simulink model "vehicles"  (Simulink 6.5)
settings: Solver=ode45  StartTime=0.0  StopTime=50  FixedStep=.1  RelTol=1e-3
PreLoadFcn:
  | vehicledata; % load in workspace variables
  | h=frontend; % bring up GUI
  | movegui(h,'northwest') % move gui to top right
PostLoadFcn:
  | rt=sfroot; chart=rt.find('-isa', 'Stateflow.Chart', '-and', 'Name','uav_modes'); chart.view;
undefined symbols (not defined in the file or in its folder): Cd0, Clmax, Clmin, g, initthis, k, magnitude, mat2cell, num_ac, num_instincts, obstacles, omega_chi, omega_gamma, omega_v, rho, S, sigma_a, sigma_o, sigma_t1, sigma_t2, targets, Tmax, W
libraries: dspmtrx3 x38, dspindex x5, dspstat3 x4, vrlib x2
(part 1 of 2)
settings Model: Creator=dlluch  LastModifiedBy=dlluch  BufferReuse=off
settings DataIOCC: LimitDataPoints=off  SaveOutput=off  SaveState=on  SignalLoggingName=sigsOut
settings OptimizationCC: BooleanDataType=off  InlineInvariantSignals=on  OptimizeBlockIOStorage=off  BufferReuse=off  ExpressionFolding=off  LocalBlockOutputs=off
settings DebuggingCC: SolverPrmCheckMsg=none  MultiTaskDSMMsg=warning  MultiTaskCondExecSysMsg=none  UnconnectedInputMsg=none  UnconnectedOutputMsg=none  UnconnectedLineMsg=none  StrictBusMsg=None
settings HardwareCC: TargetUnknown=on
settings RTWCC: IncludeERTFirstTime=on

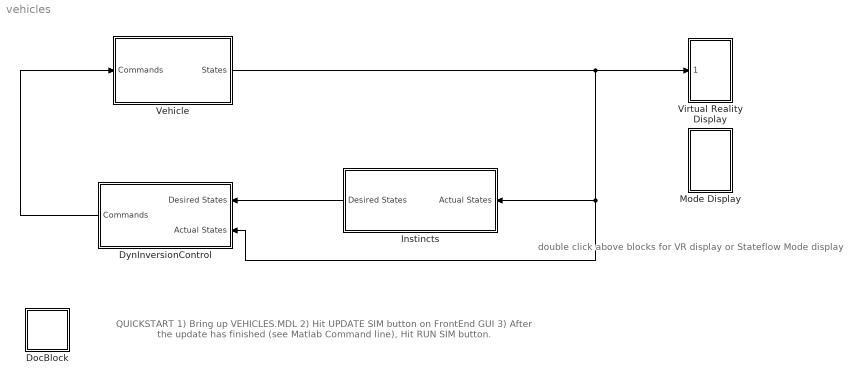
== system vehicles ==
  note: QUICKSTART
      | 1) Bring up VEHICLES.MDL
      | 2) Hit UPDATE SIM button on FrontEnd GUI
      | 3) After the update has finished (see Matlab Command line), Hit RUN SIM button.
  note: double click above
      | blocks for VR display
      | or Stateflow Mode
      | display
  DocBlock : Subsystem  mask(DocBlock){ECoderFlag=, DocumentType=Text}
      mask prompts: ECoderFlag "E Coder Flag"; DocumentType "Document Type"
      mask help: Use this block to save long descriptive text with the model. Double-clicking the block will open an editor.
      settings: CopyFcn=docblock('breaklink',gcb);  DeleteFcn=docblock('close_document',gcb);  PreSaveFcn=docblock('save_document',gcb);  OpenFcn=docblock('edit_document',gcb);
      mask StyleString: edit,popup(Text|RTF|HTML)
      mask Display:
      | plot([.8 0 0 1 1 .8 .8 1],[1 1 0 0 .8 1 .8 .8]);
      | text(.5,.5,'DOC','horizontalalignment','center');
  DynInversionControl : Subsystem  Orientation=left
  Instincts : Subsystem  Orientation=left
  Mode Display : Subsystem
      settings: OpenFcn=rt=sfroot; chart=rt.find('-isa', 'Stateflow.Chart', '-and', '-regexp', 'Name','uav_modes'); chart.view;
  Vehicle : Subsystem
  Virtual Reality Display : Subsystem
      settings: OpenFcn=|
      | h_vrsink=find_system(gcbh,'referenceblock','vrlib/VR Sink')
      | vrmfunc('FnOpen', h_vrsink);
  wires:
  Vehicle/1(States) -> Instincts/1(Actual States), DynInversionControl/2(Actual States), Virtual Reality Display/1(States)
  Instincts/1(Desired States) -> DynInversionControl/1(Desired States)
  DynInversionControl/1(Commands) -> Vehicle/1(Commands)

== system vehicles/DocBlock ==
  EmptySubsystem : Subsystem

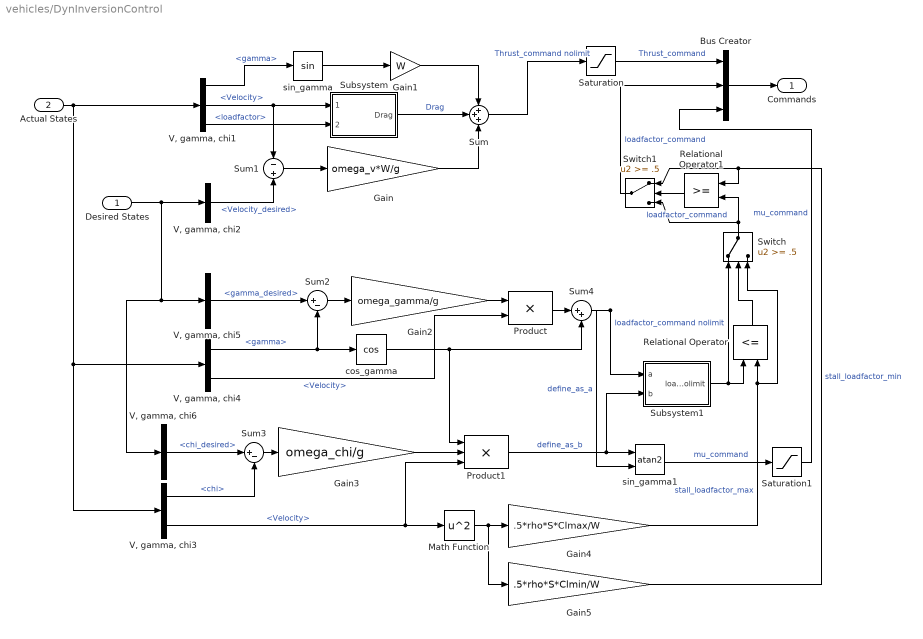
== system vehicles/DynInversionControl ==
  Desired States : Inport
  Actual States : Inport  Port=2
  Bus Creator : BusCreator  Inputs=3
  Gain : Gain  Gain=omega_v*W/g  SaturateOnIntegerOverflow=on
  Gain1 : Gain  Gain=W  SaturateOnIntegerOverflow=on
  Gain2 : Gain  Gain=omega_gamma/g  SaturateOnIntegerOverflow=on
  Gain3 : Gain  Gain=omega_chi/g  SaturateOnIntegerOverflow=on
  Gain4 : Gain  Gain=.5*rho*S*Clmax/W  SaturateOnIntegerOverflow=on
  Gain5 : Gain  Gain=.5*rho*S*Clmin/W  SaturateOnIntegerOverflow=on
  Math Function : Math  Operator=square  SaturateOnIntegerOverflow=on
  Product : Product  SaturateOnIntegerOverflow=on  InputSameDT=on
  Product1 : Product  Inputs=3  SaturateOnIntegerOverflow=on  InputSameDT=on
  Relational Operator : RelationalOperator  Orientation=up  Operator=<=  InputSameDT=on
  Relational Operator1 : RelationalOperator  Orientation=left  InputSameDT=on
  Saturation : Saturate  UpperLimit=Tmax  LowerLimit=0
  Saturation1 : Saturate  UpperLimit=pi/2  LowerLimit=-pi/2
  Subsystem : Subsystem
  Subsystem1 : Subsystem
  Sum : Sum  Inputs=+++  SaturateOnIntegerOverflow=on  InputSameDT=on
  Sum1 : Sum  Inputs=-|+  SaturateOnIntegerOverflow=on  InputSameDT=on
  Sum2 : Sum  Inputs=|+-  SaturateOnIntegerOverflow=on  InputSameDT=on
  Sum3 : Sum  Inputs=|+-  SaturateOnIntegerOverflow=on  InputSameDT=on
  Sum4 : Sum  Inputs=|++  SaturateOnIntegerOverflow=on  InputSameDT=on
  Switch : Switch  Orientation=up  Threshold=.5  SaturateOnIntegerOverflow=on  InputSameDT=on
  Switch1 : Switch  Orientation=left  Threshold=.5  SaturateOnIntegerOverflow=on  InputSameDT=on
  "V, gamma, chi1" : BusSelector  OutputSignals=gamma,Velocity,loadfactor
  "V, gamma, chi2" : BusSelector  OutputSignals=Velocity_desired
  "V, gamma, chi3" : BusSelector  OutputSignals=chi,Velocity
  "V, gamma, chi4" : BusSelector  OutputSignals=gamma,Velocity
  "V, gamma, chi5" : BusSelector  OutputSignals=gamma_desired
  "V, gamma, chi6" : BusSelector  OutputSignals=chi_desired
  cos_gamma : Trigonometry  Operator=cos
  sin_gamma : Trigonometry
  sin_gamma1 : Trigonometry  Operator=atan2
  Commands : Outport
  wires:
  Actual States/1 -> "V, gamma, chi1"/1, "V, gamma, chi3"/1, "V, gamma, chi4"/1
  "V, gamma, chi1"/3 -> Subsystem/2(loadfactor)  "<loadfactor>"
  "V, gamma, chi1"/2 -> Sum1/1, Subsystem/1(Velocity)  "<Velocity>"
  Desired States/1 -> "V, gamma, chi2"/1, "V, gamma, chi5"/1, "V, gamma, chi6"/1
  "V, gamma, chi2"/1 -> Sum1/2  "<Velocity_desired>"
  Sum1/1 -> Gain/1
  Subsystem/1(Drag) -> Sum/2  "Drag"
  Gain/1 -> Sum/3
  "V, gamma, chi1"/1 -> sin_gamma/1  "<gamma>"
  sin_gamma/1 -> Gain1/1
  Gain1/1 -> Sum/1
  Sum/1 -> Saturation/1  "Thrust_command nolimit"
  "V, gamma, chi5"/1 -> Sum2/1  "<gamma_desired>"
  "V, gamma, chi4"/1 -> Sum2/2, cos_gamma/1  "<gamma>"
  "V, gamma, chi6"/1 -> Sum3/1  "<chi_desired>"
  "V, gamma, chi3"/1 -> Sum3/2  "<chi>"
  Sum2/1 -> Gain2/1
  Gain2/1 -> Product/1
  "V, gamma, chi4"/2 -> Product/2  "<Velocity>"
  Product/1 -> Sum4/1
  cos_gamma/1 -> Sum4/2, Product1/1
  Sum4/1 -> sin_gamma1/2, Subsystem1/1(a)  "define_as_a"
  Sum3/1 -> Gain3/1
  Product1/1 -> sin_gamma1/1, Subsystem1/2(b)  "define_as_b"
  sin_gamma1/1 -> Saturation1/1  "mu_command"
  Subsystem1/1(loadfactor_nolimit) -> Switch/1, Relational Operator/1  "loadfactor_command nolimit"
  Bus Creator/1 -> Commands/1
  Saturation/1 -> Bus Creator/1  "Thrust_command"
  "V, gamma, chi3"/2 -> Product1/3, Math Function/1  "<Velocity>"
  Gain3/1 -> Product1/2
  Gain4/1 -> Switch/3, Relational Operator/2  "stall_loadfactor_max"
  Relational Operator/1 -> Switch/2
  Math Function/1 -> Gain4/1, Gain5/1
  Saturation1/1 -> Bus Creator/3  "mu_command"
  Gain5/1 -> Switch1/1, Relational Operator1/1  "stall_loadfactor_min"
  Switch/1 -> Switch1/3, Relational Operator1/2  "loadfactor_command"
  Relational Operator1/1 -> Switch1/2
  Switch1/1 -> Bus Creator/2  "loadfactor_command"

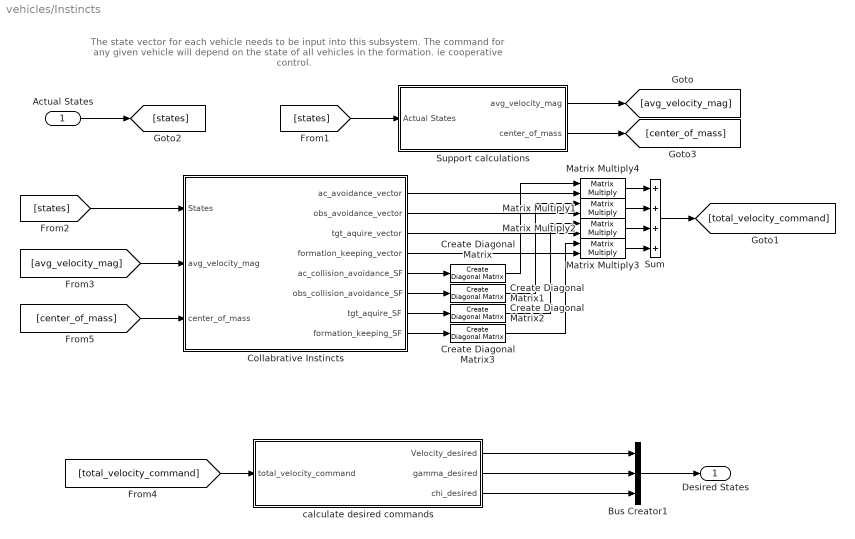
== system vehicles/Instincts ==
  note: The state vector for each vehicle needs to be input into this subsystem.  The command
      | for any given vehicle will depend on the state of all vehicles in the formation.  ie cooperative control.
  Actual States : Inport
  Bus Creator1 : BusCreator  Inputs=3
  Collabrative Instincts : Subsystem
  Create Diagonal Matrix{,1..3} (4 alike) : dspmtrx3/Create Diagonal Matrix
  Matrix Multiply{1..4} (4 alike) : Product  Multiplication=Matrix(*)
  Sum : Sum  Inputs=++++  SaturateOnIntegerOverflow=on  InputSameDT=on
  Support calculations : Subsystem
  calculate desired commands : Subsystem
  Desired States : Outport
  wires:
  Actual States/1 -> [states]
  Support calculations/1(avg_velocity_mag) -> [avg_velocity_mag]
  [states] -> Support calculations/1(Actual States)
  [states] -> Collabrative Instincts/1(States)
  [avg_velocity_mag] -> Collabrative Instincts/2(avg_velocity_mag)
  Support calculations/2(center_of_mass) -> [center_of_mass]
  [center_of_mass] -> Collabrative Instincts/3(center_of_mass)
  Collabrative Instincts/1(ac_avoidance_vector) -> Matrix Multiply4/2
  Collabrative Instincts/2(obs_avoidance_vector) -> Matrix Multiply1/2
  Collabrative Instincts/3(tgt_aquire_vector) -> Matrix Multiply2/2
  Collabrative Instincts/4(formation_keeping_vector) -> Matrix Multiply3/2
  Create Diagonal Matrix/1 -> Matrix Multiply4/1
  Create Diagonal Matrix1/1 -> Matrix Multiply1/1
  Create Diagonal Matrix2/1 -> Matrix Multiply2/1
  Collabrative Instincts/5(ac_collision_avoidance_SF) -> Create Diagonal Matrix/1
  Collabrative Instincts/6(obs_collision_avoidance_SF) -> Create Diagonal Matrix1/1
  Collabrative Instincts/7(tgt_aquire_SF) -> Create Diagonal Matrix2/1
  Collabrative Instincts/8(formation_keeping_SF) -> Create Diagonal Matrix3/1
  Matrix Multiply4/1 -> Sum/1
  Matrix Multiply1/1 -> Sum/2
  Matrix Multiply2/1 -> Sum/3
  Matrix Multiply3/1 -> Sum/4
  Create Diagonal Matrix3/1 -> Matrix Multiply3/1
  Sum/1 -> [total_velocity_command]
  [total_velocity_command] -> calculate desired commands/1(total_velocity_command)
  calculate desired commands/1(Velocity_desired) -> Bus Creator1/1
  calculate desired commands/2(gamma_desired) -> Bus Creator1/2
  calculate desired commands/3(chi_desired) -> Bus Creator1/3
  Bus Creator1/1 -> Desired States/1

== system vehicles/Mode Display ==
  Matrix Concatenation : Concatenate  NumInputs=num_instincts  Mode=Vertical matrix concatenation
  Reshape : Reshape
  Subsystem : Subsystem
  uav_modes : Stateflow chart  Orientation=up
  wires:
  Matrix Concatenation/1 -> Subsystem/1(SF)
  Subsystem/1(triggers) -> Reshape/1
  [ac_collision_avoidance_SF] -> Matrix Concatenation/1
  [obs_collision_avoidance_SF] -> Matrix Concatenation/2
  [tgt_aquire_SF] -> Matrix Concatenation/3
  [formation_keeping_SF] -> Matrix Concatenation/4
  Reshape/1 -> uav_modes/Trigger

== system vehicles/Vehicle ==
  Commands : Inport
  EOM : Subsystem
  Integrator : Integrator  InitialCondition=initthis('state_ic',num_ac)
  makebus : Subsystem
  States : Outport
  wires:
  EOM/1(State Rates) -> Integrator/1
  Integrator/1 -> makebus/1(In1)
  Commands/1 -> EOM/1(Commands)
  makebus/1(Out2) -> States/1, EOM/2(States)

== system vehicles/Virtual Reality Display ==
  note: VR coordinate system must be right hand rule.  Aircraft
      | location is (one of the) standard North-East-Up.  Therefore we will negate
      | altitude, making the resulting coor sys RHed (NED).  This will then
      | assume that the CS in the VR world is NED as well.
  States : Inport
  Gain1 : Gain  Gain=-1  SaturateOnIntegerOverflow=on
  Multiport Selector : dspindex/Multiport Selector  rowsOrCols=Rows  idxCellArray=mat2cell(1:num_ac,1,ones(1,num_ac))  idxErrMode=Clip Index
  VR Placeholder : vrlib/VR Placeholder  SystemSampleTime=-1  outwidth=4
  VR Sink : vrlib/VR Sink  SampleTime=0.5  ViewEnable=on  RemoteChange=off  RemoteView=off  FieldsWritten=uav1.rotation#uav1.translation#uav2.rotation#uav2.translation#uav3.rotation#uav3.translation#uav4.rotation#uav4.translation#uav5.rotation#uav5.translation  WorldFileName=temp.wrl  WorldDescription=Multiple UAV Simulation  AutoView=off  FigureProperties={}
  positions of each AC : Concatenate  NumInputs=3  Mode=Horizontal matrix concatenation
  x,y,h : BusSelector  OutputSignals=x,y,h
  wires:
  States/1 -> x,y,h/1
  x,y,h/3 -> Gain1/1  "<h>"
  x,y,h/2 -> positions of each AC/2  "<y>"
  x,y,h/1 -> positions of each AC/1  "<x>"
  positions of each AC/1 -> Multiport Selector/1
  Gain1/1 -> positions of each AC/3
  Multiport Selector/1 -> VR Sink/2
  Multiport Selector/2 -> VR Sink/4
  Multiport Selector/3 -> VR Sink/6
  Multiport Selector/4 -> VR Sink/8
  Multiport Selector/5 -> VR Sink/10
  VR Placeholder/1 -> VR Sink/1, VR Sink/3, VR Sink/5, VR Sink/7, VR Sink/9

== system vehicles/DocBlock/EmptySubsystem ==

== system vehicles/DynInversionControl/Subsystem ==
  Velocity : Inport
  loadfactor : Inport  Port=2
  Constant : Constant  Value=Cd0  OutDataType=sfix(16)  ConRadixGroup=Use specified scaling  OutScaling=2^0  SampleTime=inf  FramePeriod=inf
  Gain1 : Gain  Gain=2*W/(rho*S)  SaturateOnIntegerOverflow=on
  Gain3 : Gain  Gain=k  SaturateOnIntegerOverflow=on
  Gain4 : Gain  Gain=.5*rho*S  SaturateOnIntegerOverflow=on
  Math Function : Math  Operator=square  SaturateOnIntegerOverflow=on
  Math Function2 : Math  Operator=square  SaturateOnIntegerOverflow=on
  Product1 : Product  Inputs=/*  SaturateOnIntegerOverflow=on  InputSameDT=on
  Product2 : Product  SaturateOnIntegerOverflow=on  InputSameDT=on
  Sum1 : Sum  Inputs=|++  SaturateOnIntegerOverflow=on  InputSameDT=on
  Drag : Outport
  wires:
  Velocity/1 -> Math Function/1
  loadfactor/1 -> Gain1/1
  Math Function/1 -> Product2/1, Product1/1
  Product1/1 -> Math Function2/1  "Cl"
  Math Function2/1 -> Gain3/1
  Gain3/1 -> Sum1/1
  Constant/1 -> Sum1/2
  Sum1/1 -> Gain4/1
  Gain4/1 -> Product2/2
  Product2/1 -> Drag/1
  Gain1/1 -> Product1/2

== system vehicles/DynInversionControl/Subsystem1 ==
  a : Inport
  b : Inport  Port=2
  Math Function : Math  Operator=square  SaturateOnIntegerOverflow=on
  Math Function1 : Math  Operator=square  SaturateOnIntegerOverflow=on
  Math Function2 : Math  Operator=sqrt  SaturateOnIntegerOverflow=on
  Sum : Sum  Inputs=|++  SaturateOnIntegerOverflow=on  InputSameDT=on
  loadfactor_nolimit : Outport
  wires:
  Math Function2/1 -> loadfactor_nolimit/1
  Math Function1/1 -> Sum/2
  Math Function/1 -> Sum/1
  b/1 -> Math Function1/1
  a/1 -> Math Function/1
  Sum/1 -> Math Function2/1

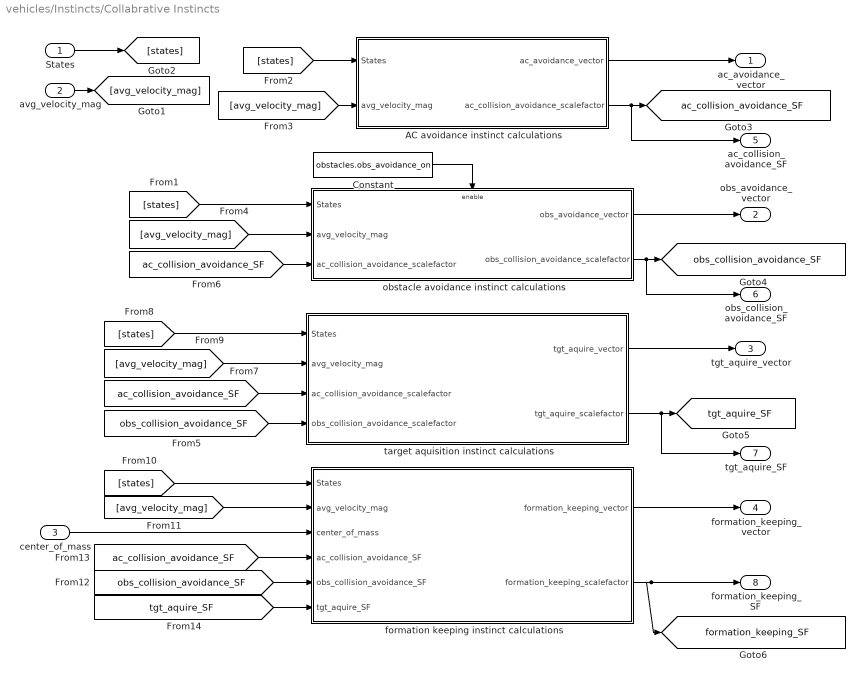
== system vehicles/Instincts/Collabrative Instincts ==
  States : Inport
  avg_velocity_mag : Inport  Port=2
  center_of_mass : Inport  Port=3
  AC avoidance instinct calculations : Subsystem
  Constant : Constant  Value=obstacles.obs_avoidance_on  OutDataType=sfix(16)  ConRadixGroup=Use specified scaling  OutScaling=2^0  SampleTime=inf  FramePeriod=inf
  formation keeping instinct calculations : Subsystem
  obstacle avoidance instinct calculations : Subsystem  TreatAsAtomicUnit=on
  target aquisition instinct calculations : Subsystem
  ac_avoidance_vector : Outport
  obs_avoidance_vector : Outport  Port=2
  tgt_aquire_vector : Outport  Port=3
  formation_keeping_vector : Outport  Port=4
  ac_collision_avoidance_SF : Outport  Port=5
  obs_collision_avoidance_SF : Outport  Port=6
  tgt_aquire_SF : Outport  Port=7
  formation_keeping_SF : Outport  Port=8
  tag scope: ac_collision_avoidance_SF=global, formation_keeping_SF=global, obs_collision_avoidance_SF=global, tgt_aquire_SF=global
  wires:
  Constant/1 -> obstacle avoidance instinct calculations/Enable
  AC avoidance instinct calculations/2(ac_collision_avoidance_scalefactor) -> [ac_collision_avoidance_SF], ac_collision_avoidance_SF/1
  AC avoidance instinct calculations/1(ac_avoidance_vector) -> ac_avoidance_vector/1
  obstacle avoidance instinct calculations/1(obs_avoidance_vector) -> obs_avoidance_vector/1
  obstacle avoidance instinct calculations/2(obs_collision_avoidance_scalefactor) -> [obs_collision_avoidance_SF], obs_collision_avoidance_SF/1
  [ac_collision_avoidance_SF] -> obstacle avoidance instinct calculations/3(ac_collision_avoidance_scalefactor)
  [states] -> obstacle avoidance instinct calculations/1(States)
  [states] -> AC avoidance instinct calculations/1(States)
  States/1 -> [states]
  avg_velocity_mag/1 -> [avg_velocity_mag]
  [avg_velocity_mag] -> AC avoidance instinct calculations/2(avg_velocity_mag)
  [avg_velocity_mag] -> obstacle avoidance instinct calculations/2(avg_velocity_mag)
  [states] -> target aquisition instinct calculations/1(States)
  [obs_collision_avoidance_SF] -> target aquisition instinct calculations/4(obs_collision_avoidance_scalefactor)
  [ac_collision_avoidance_SF] -> target aquisition instinct calculations/3(ac_collision_avoidance_scalefactor)
  [avg_velocity_mag] -> target aquisition instinct calculations/2(avg_velocity_mag)
  target aquisition instinct calculations/1(tgt_aquire_vector) -> tgt_aquire_vector/1
  target aquisition instinct calculations/2(tgt_aquire_scalefactor) -> [tgt_aquire_SF], tgt_aquire_SF/1
  [states] -> formation keeping instinct calculations/1(States)
  center_of_mass/1 -> formation keeping instinct calculations/3(center_of_mass)
  [avg_velocity_mag] -> formation keeping instinct calculations/2(avg_velocity_mag)
  [ac_collision_avoidance_SF] -> formation keeping instinct calculations/4(ac_collision_avoidance_SF)
  [obs_collision_avoidance_SF] -> formation keeping instinct calculations/5(obs_collision_avoidance_SF)
  [tgt_aquire_SF] -> formation keeping instinct calculations/6(tgt_aquire_SF)
  formation keeping instinct calculations/2(formation_keeping_scalefactor) -> formation_keeping_SF/1, [formation_keeping_SF]
  formation keeping instinct calculations/1(formation_keeping_vector) -> formation_keeping_vector/1

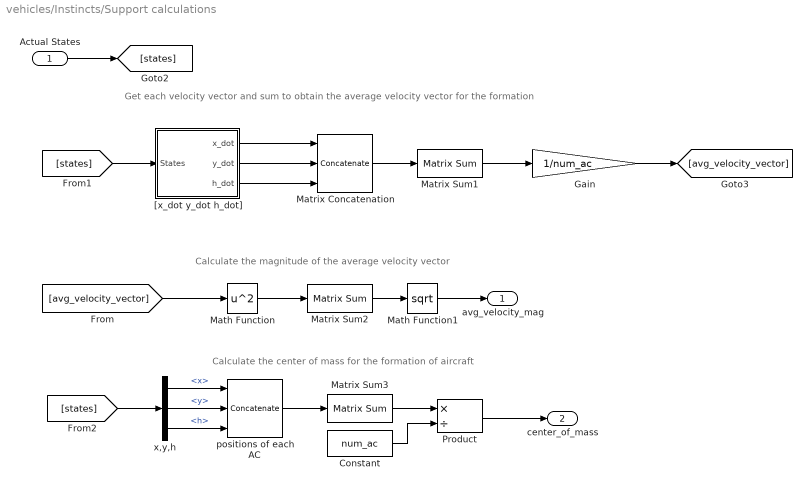
== system vehicles/Instincts/Support calculations ==
  note: Calculate the magnitude of the average velocity vector
  note: Calculate the center of mass for the formation of aircraft
  note: Get each velocity vector and sum to obtain the average velocity vector for the formation
  Actual States : Inport
  Constant : Constant  Value=num_ac  OutDataType=sfix(16)  ConRadixGroup=Use specified scaling  OutScaling=2^0  SampleTime=inf  FramePeriod=inf
  Gain : Gain  Gain=1/num_ac  SaturateOnIntegerOverflow=on
  Math Function : Math  Operator=square  SaturateOnIntegerOverflow=on
  Math Function1 : Math  Operator=sqrt  SaturateOnIntegerOverflow=on
  Matrix Concatenation : Concatenate  NumInputs=3  Mode=Horizontal matrix concatenation
  Matrix Sum1 : dspmtrx3/Matrix Sum  DialogController=dspDDGCreate  DialogControllerArgs=DataTag24  Dim=Columns  roundingMode=Floor  overflowMode=off
  Matrix Sum2 : dspmtrx3/Matrix Sum  DialogController=dspDDGCreate  DialogControllerArgs=DataTag25  Dim=Rows  roundingMode=Floor  overflowMode=off
  Matrix Sum3 : dspmtrx3/Matrix Sum  DialogController=dspDDGCreate  DialogControllerArgs=DataTag26  Dim=Columns  roundingMode=Floor  overflowMode=off
  Product : Product  Inputs=*/  SaturateOnIntegerOverflow=on  InputSameDT=on
  "[x_dot y_dot h_dot]" : Subsystem
  positions of each AC : Concatenate  NumInputs=3  Mode=Horizontal matrix concatenation
  x,y,h : BusSelector  OutputSignals=x,y,h
  avg_velocity_mag : Outport
  center_of_mass : Outport  Port=2
  wires:
  "[x_dot y_dot h_dot]"/1(x_dot) -> Matrix Concatenation/1
  "[x_dot y_dot h_dot]"/2(y_dot) -> Matrix Concatenation/2
  "[x_dot y_dot h_dot]"/3(h_dot) -> Matrix Concatenation/3
  Matrix Concatenation/1 -> Matrix Sum1/1
  Matrix Sum1/1 -> Gain/1
  [avg_velocity_vector] -> Math Function/1
  Math Function/1 -> Matrix Sum2/1
  Matrix Sum2/1 -> Math Function1/1
  Math Function1/1 -> avg_velocity_mag/1
  x,y,h/1 -> positions of each AC/1  "<x>"
  x,y,h/2 -> positions of each AC/2  "<y>"
  x,y,h/3 -> positions of each AC/3  "<h>"
  positions of each AC/1 -> Matrix Sum3/1
  Matrix Sum3/1 -> Product/1
  Constant/1 -> Product/2
  Gain/1 -> [avg_velocity_vector]
  [states] -> x,y,h/1
  Product/1 -> center_of_mass/1
  Actual States/1 -> [states]
  [states] -> "[x_dot y_dot h_dot]"/1(States)

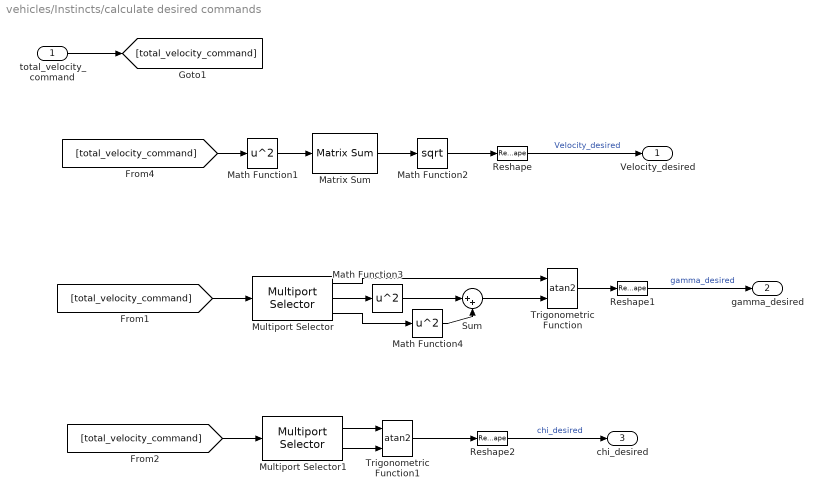
== system vehicles/Instincts/calculate desired commands ==
  total_velocity_command : Inport
  Math Function1 : Math  Operator=square  SaturateOnIntegerOverflow=on
  Math Function2 : Math  Operator=sqrt  SaturateOnIntegerOverflow=on
  Math Function3 : Math  Operator=square  SaturateOnIntegerOverflow=on
  Math Function4 : Math  Operator=square  SaturateOnIntegerOverflow=on
  Matrix Sum : dspmtrx3/Matrix Sum  DialogController=dspDDGCreate  DialogControllerArgs=DataTag27  Dim=Rows  roundingMode=Floor  overflowMode=off
  Multiport Selector : dspindex/Multiport Selector  rowsOrCols=Columns  idxCellArray={3, 1, 2}  idxErrMode=Clip Index
  Multiport Selector1 : dspindex/Multiport Selector  rowsOrCols=Columns  idxCellArray={2,1}  idxErrMode=Clip Index
  Reshape : Reshape
  Reshape1 : Reshape
  Reshape2 : Reshape
  Sum : Sum  Inputs=|++  SaturateOnIntegerOverflow=on  InputSameDT=on
  Trigonometric Function : Trigonometry  Operator=atan2
  Trigonometric Function1 : Trigonometry  Operator=atan2
  Velocity_desired : Outport
  gamma_desired : Outport  Port=2
  chi_desired : Outport  Port=3
  wires:
  Math Function1/1 -> Matrix Sum/1
  Matrix Sum/1 -> Math Function2/1
  Math Function2/1 -> Reshape/1
  Reshape/1 -> Velocity_desired/1  "Velocity_desired"
  total_velocity_command/1 -> [total_velocity_command]
  [total_velocity_command] -> Math Function1/1
  [total_velocity_command] -> Multiport Selector/1
  Math Function3/1 -> Sum/1
  Math Function4/1 -> Sum/2
  Trigonometric Function/1 -> Reshape1/1
  [total_velocity_command] -> Multiport Selector1/1
  Multiport Selector1/1 -> Trigonometric Function1/1
  Multiport Selector1/2 -> Trigonometric Function1/2
  Trigonometric Function1/1 -> Reshape2/1
  Reshape1/1 -> gamma_desired/1  "gamma_desired"
  Reshape2/1 -> chi_desired/1  "chi_desired"
  Multiport Selector/2 -> Math Function3/1
  Multiport Selector/3 -> Math Function4/1
  Multiport Selector/1 -> Trigonometric Function/1
  Sum/1 -> Trigonometric Function/2

== system vehicles/Mode Display/Subsystem ==
  note: this subsystem will make the triggers for the stateflow machine.
      | This will output a [number of instincts x number of aircraft] matrix.
      | each column will have a single value of unity on the instint that is
      | winning.
  SF : Inport
  Constant1 : Constant  Value=ones(num_instincts,1)  VectorParams1D=off  OutDataType=sfix(16)  ConRadixGroup=Use specified scaling  OutScaling=2^0  SampleTime=inf  FramePeriod=inf
  Matrix Multiply : Product  Multiplication=Matrix(*)
  Maximum of columns : dspstat3/Maximum  DialogController=dspfixptddg.MinMax  DialogControllerArgs=DataTag28  fcn=Value  reset=None  indexBase=One  operateOver=Each column  colComp=on  operation=maximum  roundingMode=Floor  overflowMode=off
  Relational Operator : RelationalOperator  Operator===  InputSameDT=on
  triggers : Outport
  wires:
  SF/1 -> Relational Operator/1, Maximum of columns/1
  Maximum of columns/1 -> Matrix Multiply/2
  Constant1/1 -> Matrix Multiply/1
  Matrix Multiply/1 -> Relational Operator/2
  Relational Operator/1 -> triggers/1

== system vehicles/Vehicle/EOM ==
  Commands : Inport
  States : Inport  Port=2
  Matrix Concatenation : Concatenate  NumInputs=9  Mode=Horizontal matrix concatenation
  Transpose : dspmtrx3/Transpose  SystemSampleTime=-1  Hermitian=off  overflowFlag=on
  "[Velocity_dot gamma_dot chi_dot]" : Subsystem
  "[thrust_dot mu_dot loadfactor_dot]" : Subsystem
  "[x_dot y_dot h_dot]" : Subsystem
  State Rates : Outport
  wires:
  Commands/1 -> "[thrust_dot mu_dot loadfactor_dot]"/1(Comands), "[Velocity_dot gamma_dot chi_dot]"/2(Commands)
  States/1 -> "[Velocity_dot gamma_dot chi_dot]"/1(States), "[thrust_dot mu_dot loadfactor_dot]"/2(States), "[x_dot y_dot h_dot]"/1(States)
  "[x_dot y_dot h_dot]"/1(x_dot) -> Matrix Concatenation/7
  "[x_dot y_dot h_dot]"/2(y_dot) -> Matrix Concatenation/8
  "[x_dot y_dot h_dot]"/3(h_dot) -> Matrix Concatenation/9
  "[Velocity_dot gamma_dot chi_dot]"/2(gamma_dot) -> Matrix Concatenation/2
  "[Velocity_dot gamma_dot chi_dot]"/1(Velocity_dot) -> Matrix Concatenation/1
  "[Velocity_dot gamma_dot chi_dot]"/3(chi_dot) -> Matrix Concatenation/3
  "[thrust_dot mu_dot loadfactor_dot]"/2(mu_dot) -> Matrix Concatenation/5
  "[thrust_dot mu_dot loadfactor_dot]"/1(thrust_dot) -> Matrix Concatenation/4
  "[thrust_dot mu_dot loadfactor_dot]"/3(loadfactor_dot) -> Matrix Concatenation/6
  Transpose/1 -> State Rates/1
  Matrix Concatenation/1 -> Transpose/1

== system vehicles/Vehicle/makebus ==
  In1 : Inport  PortDimensions=[9,num_ac]
  Bus Creator : BusCreator  Inputs=9
  Multiport Selector : dspindex/Multiport Selector  rowsOrCols=Rows  idxCellArray={ 1,2,3,4,5,6,7,8,9}  idxErrMode=Clip Index
  Reshape{,1..8} (9 alike) : Reshape
  Out2 : Outport
  wires:
  Multiport Selector/1 -> Reshape/1  "Velocity"
  Multiport Selector/2 -> Reshape1/1  "gamma"
  Multiport Selector/3 -> Reshape2/1  "chi"
  Multiport Selector/4 -> Reshape3/1  "thrust"
  Multiport Selector/5 -> Reshape4/1  "mu"
  Multiport Selector/6 -> Reshape5/1  "loadfactor"
  Multiport Selector/7 -> Reshape6/1  "x"
  Multiport Selector/8 -> Reshape7/1  "y"
  Multiport Selector/9 -> Reshape8/1  "h"
  In1/1 -> Multiport Selector/1
  Bus Creator/1 -> Out2/1
  Reshape/1 -> Bus Creator/1  "Velocity"
  Reshape1/1 -> Bus Creator/2  "gamma"
  Reshape2/1 -> Bus Creator/3  "chi"
  Reshape3/1 -> Bus Creator/4  "thrust"
  Reshape4/1 -> Bus Creator/5  "mu"
  Reshape5/1 -> Bus Creator/6  "loadfactor"
  Reshape6/1 -> Bus Creator/7  "x"
  Reshape7/1 -> Bus Creator/8  "y"
  Reshape8/1 -> Bus Creator/9  "h"

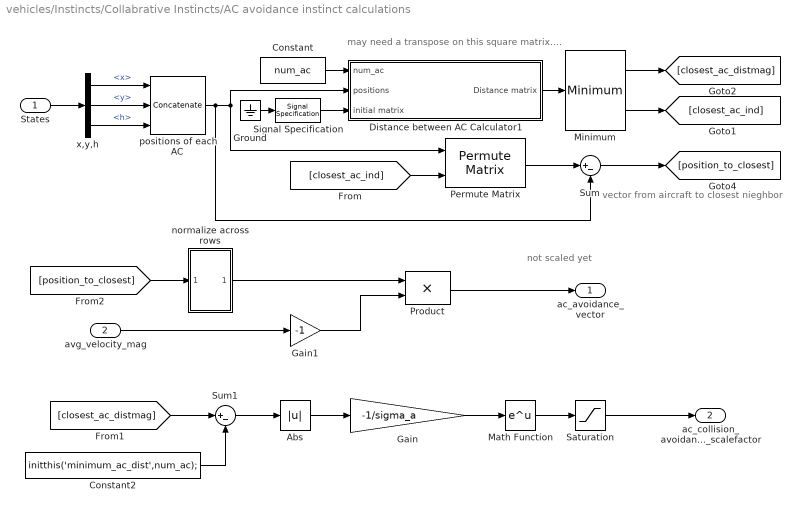
== system vehicles/Instincts/Collabrative Instincts/AC avoidance instinct calculations ==
  note: vector from aircraft to closest nieghbor
  note: may need a transpose on this square matrix....
  note: not scaled yet
  States : Inport
  avg_velocity_mag : Inport  Port=2
  Abs : Abs  SaturateOnIntegerOverflow=on  SampleTime=-1
  Constant : Constant  Value=num_ac  OutDataType=sfix(16)  ConRadixGroup=Use specified scaling  OutScaling=2^0  SampleTime=inf  FramePeriod=inf
  Constant2 : Constant  Value=initthis('minimum_ac_dist',num_ac);  OutDataType=sfix(16)  ConRadixGroup=Use specified scaling  OutScaling=2^0  SampleTime=inf  FramePeriod=inf
  Distance between AC Calculator1 : Subsystem  TreatAsAtomicUnit=on
  Gain : Gain  Gain=-1/sigma_a  SaturateOnIntegerOverflow=on
  Gain1 : Gain  Gain=-1  SaturateOnIntegerOverflow=on
  Ground : Ground
  Math Function : Math  SaturateOnIntegerOverflow=on
  Minimum : dspstat3/Minimum  DialogController=dspfixptddg.MinMax  DialogControllerArgs=DataTag2  fcn=Value and Index  reset=None  indexBase=One  operateOver=Each column  colComp=on  operation=minimum  roundingMode=Floor  overflowMode=off
  Permute Matrix : dspmtrx3/Permute Matrix  mode=Rows  ZeroOneIdxMode=One-based  errmode=Clip index  checkDims=off
  Product : Product  SaturateOnIntegerOverflow=on  InputSameDT=on
  Saturation : Saturate  UpperLimit=1  LowerLimit=0
  Signal Specification : SignalSpecification  Dimensions=[num_ac,num_ac]
  Sum : Sum  Inputs=|+-  SaturateOnIntegerOverflow=on  InputSameDT=on
  Sum1 : Sum  Inputs=|+-  SaturateOnIntegerOverflow=on  InputSameDT=on
  normalize across rows : Subsystem  TreatAsAtomicUnit=on
  positions of each AC : Concatenate  NumInputs=3  Mode=Horizontal matrix concatenation
  x,y,h : BusSelector  OutputSignals=x,y,h
  ac_avoidance_vector : Outport
  ac_collision_avoidance_scalefactor : Outport  Port=2
  wires:
  States/1 -> x,y,h/1
  x,y,h/1 -> positions of each AC/1  "<x>"
  x,y,h/2 -> positions of each AC/2  "<y>"
  x,y,h/3 -> positions of each AC/3  "<h>"
  positions of each AC/1 -> Permute Matrix/1, Distance between AC Calculator1/2(positions), Sum/2
  Constant/1 -> Distance between AC Calculator1/1(num_ac)
  Distance between AC Calculator1/1(Distance matrix) -> Minimum/1
  Minimum/2 -> [closest_ac_ind]
  [closest_ac_ind] -> Permute Matrix/2
  Permute Matrix/1 -> Sum/1
  Sum/1 -> [position_to_closest]
  Minimum/1 -> [closest_ac_distmag]
  [closest_ac_distmag] -> Sum1/1
  Constant2/1 -> Sum1/2
  Sum1/1 -> Abs/1
  Gain/1 -> Math Function/1
  Math Function/1 -> Saturation/1
  [position_to_closest] -> normalize across rows/1(In1)
  normalize across rows/1(Out1) -> Product/1
  avg_velocity_mag/1 -> Gain1/1
  Gain1/1 -> Product/2
  Product/1 -> ac_avoidance_vector/1
  Abs/1 -> Gain/1
  Saturation/1 -> ac_collision_avoidance_scalefactor/1
  Ground/1 -> Signal Specification/1
  Signal Specification/1 -> Distance between AC Calculator1/3(initial matrix)

== system vehicles/Instincts/Collabrative Instincts/formation keeping instinct calculations ==
  States : Inport
  avg_velocity_mag : Inport  Port=2
  center_of_mass : Inport  Port=3
  ac_collision_avoidance_SF : Inport  Port=4
  obs_collision_avoidance_SF : Inport  Port=5
  tgt_aquire_SF : Inport  Port=6
  Constant : Constant  Value=ones(num_ac,1)  VectorParams1D=off  OutDataType=sfix(16)  ConRadixGroup=Use specified scaling  OutScaling=2^0  SampleTime=inf  FramePeriod=inf
  Constant1 : Constant  Value=1  OutDataType=sfix(16)  ConRadixGroup=Use specified scaling  OutScaling=2^0  SampleTime=inf  FramePeriod=inf
  Matrix Multiply : Product  Multiplication=Matrix(*)
  Product : Product  SaturateOnIntegerOverflow=on  InputSameDT=on
  Sum : Sum  Inputs=|-+  SaturateOnIntegerOverflow=on  InputSameDT=on
  Sum1 : Sum  Inputs=+---  SaturateOnIntegerOverflow=on  InputSameDT=on
  normalize across rows : Subsystem
  positions of each AC : Concatenate  NumInputs=3  Mode=Horizontal matrix concatenation
  x,y,h : BusSelector  OutputSignals=x,y,h
  formation_keeping_vector : Outport
  formation_keeping_scalefactor : Outport  Port=2
  wires:
  States/1 -> x,y,h/1
  x,y,h/1 -> positions of each AC/1  "<x>"
  x,y,h/2 -> positions of each AC/2  "<y>"
  x,y,h/3 -> positions of each AC/3  "<h>"
  positions of each AC/1 -> Sum/1
  Matrix Multiply/1 -> Sum/2
  Constant/1 -> Matrix Multiply/1
  center_of_mass/1 -> Matrix Multiply/2
  Sum/1 -> normalize across rows/1(In1)
  normalize across rows/1(Out1) -> Product/1
  avg_velocity_mag/1 -> Product/2
  Product/1 -> formation_keeping_vector/1
  Constant1/1 -> Sum1/1
  ac_collision_avoidance_SF/1 -> Sum1/2
  obs_collision_avoidance_SF/1 -> Sum1/3
  tgt_aquire_SF/1 -> Sum1/4
  Sum1/1 -> formation_keeping_scalefactor/1

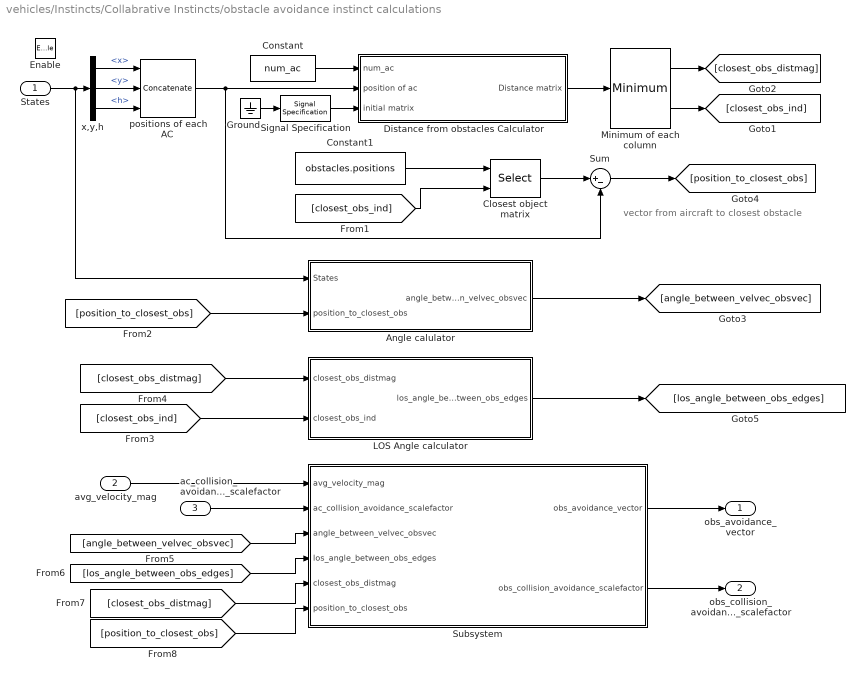
== system vehicles/Instincts/Collabrative Instincts/obstacle avoidance instinct calculations ==
  note: vector from aircraft to closest obstacle
  States : Inport
  avg_velocity_mag : Inport  Port=2
  ac_collision_avoidance_scalefactor : Inport  Port=3
  Enable : EnablePort
  Angle calulator : Subsystem
  Closest object matrix : Selector  InputType=Matrix  ElementSrc=Internal  Elements=[1 3]  RowSrc=External  Rows=1  ColumnSrc=Internal  Columns=-1  InputPortWidth=3  IndexIsStartValue=off
  Constant : Constant  Value=num_ac  OutDataType=sfix(16)  ConRadixGroup=Use specified scaling  OutScaling=2^0  SampleTime=inf  FramePeriod=inf
  Constant1 : Constant  Value=obstacles.positions  OutDataType=sfix(16)  ConRadixGroup=Use specified scaling  OutScaling=2^0  SampleTime=inf  FramePeriod=inf
  Distance from obstacles Calculator : Subsystem  TreatAsAtomicUnit=on
  Ground : Ground
  LOS Angle calculator : Subsystem
  Minimum of each column : dspstat3/Minimum  DialogController=dspfixptddg.MinMax  DialogControllerArgs=DataTag12  fcn=Value and Index  reset=None  indexBase=One  operateOver=Each column  colComp=on  operation=minimum  roundingMode=Floor  overflowMode=off
  Signal Specification : SignalSpecification  Dimensions=[size(obstacles.positions,1),num_ac]
  Subsystem : Subsystem
  Sum : Sum  Inputs=|+-  SaturateOnIntegerOverflow=on  InputSameDT=on
  positions of each AC : Concatenate  NumInputs=3  Mode=Horizontal matrix concatenation
  x,y,h : BusSelector  OutputSignals=x,y,h
  obs_avoidance_vector : Outport
  obs_collision_avoidance_scalefactor : Outport  Port=2
  wires:
  Minimum of each column/1 -> [closest_obs_distmag]
  Sum/1 -> [position_to_closest_obs]
  Minimum of each column/2 -> [closest_obs_ind]
  Distance from obstacles Calculator/1(Distance matrix) -> Minimum of each column/1
  Constant/1 -> Distance from obstacles Calculator/1(num_ac)
  positions of each AC/1 -> Sum/2, Distance from obstacles Calculator/2(position of ac)
  x,y,h/3 -> positions of each AC/3  "<h>"
  x,y,h/2 -> positions of each AC/2  "<y>"
  x,y,h/1 -> positions of each AC/1  "<x>"
  States/1 -> x,y,h/1, Angle calulator/1(States)
  [closest_obs_ind] -> Closest object matrix/2
  Constant1/1 -> Closest object matrix/1
  Closest object matrix/1 -> Sum/1
  [position_to_closest_obs] -> Angle calulator/2(position_to_closest_obs)
  Angle calulator/1(angle_between_velvec_obsvec) -> [angle_between_velvec_obsvec]
  [closest_obs_ind] -> LOS Angle calculator/2(closest_obs_ind)
  [closest_obs_distmag] -> LOS Angle calculator/1(closest_obs_distmag)
  LOS Angle calculator/1(los_angle_between_obs_edges) -> [los_angle_between_obs_edges]
  Subsystem/2(obs_collision_avoidance_scalefactor) -> obs_collision_avoidance_scalefactor/1
  avg_velocity_mag/1 -> Subsystem/1(avg_velocity_mag)
  ac_collision_avoidance_scalefactor/1 -> Subsystem/2(ac_collision_avoidance_scalefactor)
  [angle_between_velvec_obsvec] -> Subsystem/3(angle_between_velvec_obsvec)
  [los_angle_between_obs_edges] -> Subsystem/4(los_angle_between_obs_edges)
  [closest_obs_distmag] -> Subsystem/5(closest_obs_distmag)
  [position_to_closest_obs] -> Subsystem/6(position_to_closest_obs)
  Subsystem/1(obs_avoidance_vector) -> obs_avoidance_vector/1
  Signal Specification/1 -> Distance from obstacles Calculator/3(initial matrix)
  Ground/1 -> Signal Specification/1

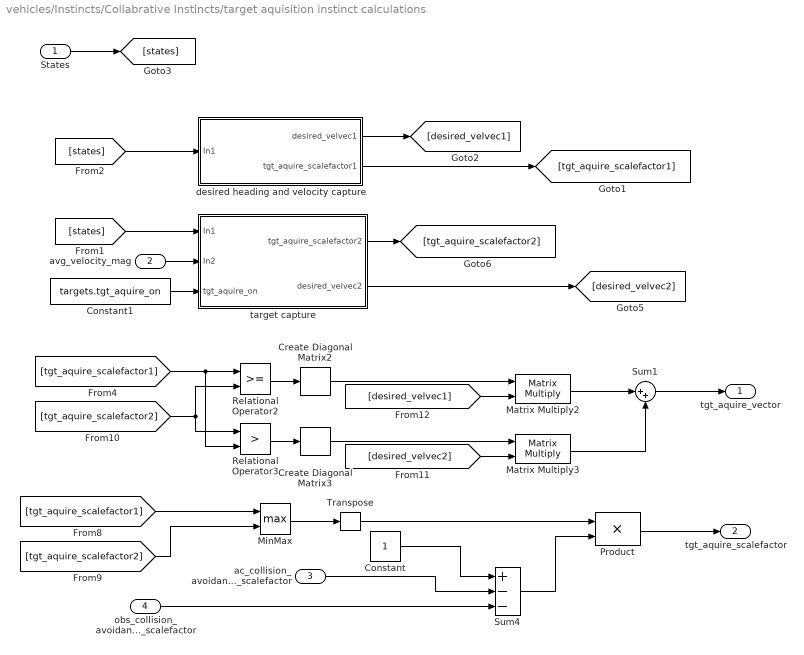
== system vehicles/Instincts/Collabrative Instincts/target aquisition instinct calculations ==
  States : Inport
  avg_velocity_mag : Inport  Port=2
  ac_collision_avoidance_scalefactor : Inport  Port=3
  obs_collision_avoidance_scalefactor : Inport  Port=4
  Constant : Constant  Value=1  OutDataType=sfix(16)  ConRadixGroup=Use specified scaling  OutScaling=2^0  SampleTime=inf  FramePeriod=inf
  Constant1 : Constant  Value=targets.tgt_aquire_on  OutDataType=sfix(16)  ConRadixGroup=Use specified scaling  OutScaling=2^0  SampleTime=inf  FramePeriod=inf
  Create Diagonal Matrix2 : dspmtrx3/Create Diagonal Matrix
  Create Diagonal Matrix3 : dspmtrx3/Create Diagonal Matrix
  Matrix Multiply2 : Product  Multiplication=Matrix(*)
  Matrix Multiply3 : Product  Multiplication=Matrix(*)
  MinMax : MinMax  Function=max  Inputs=2  SaturateOnIntegerOverflow=on  InputSameDT=on
  Product : Product  SaturateOnIntegerOverflow=on  InputSameDT=on
  Relational Operator2 : RelationalOperator  InputSameDT=on
  Relational Operator3 : RelationalOperator  Operator=>  InputSameDT=on
  Sum1 : Sum  Inputs=|++  SaturateOnIntegerOverflow=on  InputSameDT=on
  Sum4 : Sum  Inputs=+--  SaturateOnIntegerOverflow=on  InputSameDT=on
  Transpose : dspmtrx3/Transpose  SystemSampleTime=-1  Hermitian=off  overflowFlag=on
  desired heading and velocity capture : Subsystem
  target capture : Subsystem
  tgt_aquire_vector : Outport
  tgt_aquire_scalefactor : Outport  Port=2
  wires:
  desired heading and velocity capture/2(tgt_aquire_scalefactor1) -> [tgt_aquire_scalefactor1]
  States/1 -> [states]
  [states] -> target capture/1(In1)
  [states] -> desired heading and velocity capture/1(In1)
  target capture/2(desired_velvec2) -> [desired_velvec2]
  avg_velocity_mag/1 -> target capture/2(In2)
  target capture/1(tgt_aquire_scalefactor2) -> [tgt_aquire_scalefactor2]
  [tgt_aquire_scalefactor1] -> MinMax/1
  [tgt_aquire_scalefactor2] -> MinMax/2
  MinMax/1 -> Transpose/1
  ac_collision_avoidance_scalefactor/1 -> Sum4/2
  obs_collision_avoidance_scalefactor/1 -> Sum4/3
  desired heading and velocity capture/1(desired_velvec1) -> [desired_velvec1]
  Constant1/1 -> target capture/3(tgt_aquire_on)
  [tgt_aquire_scalefactor1] -> Relational Operator2/1, Relational Operator3/2
  [tgt_aquire_scalefactor2] -> Relational Operator2/2, Relational Operator3/1
  Relational Operator2/1 -> Create Diagonal Matrix2/1
  Relational Operator3/1 -> Create Diagonal Matrix3/1
  [desired_velvec1] -> Matrix Multiply2/2
  [desired_velvec2] -> Matrix Multiply3/2
  Matrix Multiply2/1 -> Sum1/1
  Matrix Multiply3/1 -> Sum1/2
  Sum1/1 -> tgt_aquire_vector/1
  Create Diagonal Matrix2/1 -> Matrix Multiply2/1
  Create Diagonal Matrix3/1 -> Matrix Multiply3/1
  Constant/1 -> Sum4/1
  Product/1 -> tgt_aquire_scalefactor/1
  Sum4/1 -> Product/2
  Transpose/1 -> Product/1

== system vehicles/Instincts/Support calculations/[x_dot y_dot h_dot] ==
  States : Inport
  Product : Product  Inputs=3  SaturateOnIntegerOverflow=on  InputSameDT=on
  Product1 : Product  SaturateOnIntegerOverflow=on  InputSameDT=on
  Product2 : Product  Inputs=3  SaturateOnIntegerOverflow=on  InputSameDT=on
  "V, gamma, chi" : BusSelector  OutputSignals=Velocity,gamma,chi
  cos_chi : Trigonometry  Operator=cos
  cos_gamma : Trigonometry  Operator=cos
  sin_chi : Trigonometry
  sin_gamma : Trigonometry
  x_dot : Outport
  y_dot : Outport  Port=2
  h_dot : Outport  Port=3
  wires:
  "V, gamma, chi"/1 -> Product2/1, Product/1, Product1/1  "<Velocity>"
  "V, gamma, chi"/2 -> sin_gamma/1, cos_gamma/1  "<gamma>"
  "V, gamma, chi"/3 -> sin_chi/1, cos_chi/1  "<chi>"
  cos_gamma/1 -> Product2/2, Product/2
  cos_chi/1 -> Product2/3
  sin_chi/1 -> Product/3
  sin_gamma/1 -> Product1/2
  States/1 -> "V, gamma, chi"/1
  Product2/1 -> x_dot/1  "x_dot"
  Product/1 -> y_dot/1  "y_dot"
  Product1/1 -> h_dot/1  "h_dot"

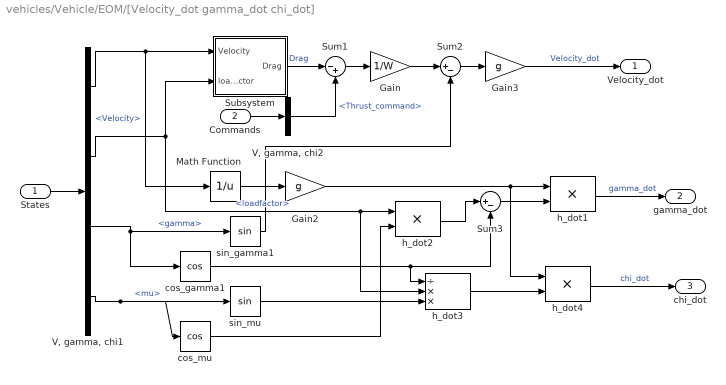
== system vehicles/Vehicle/EOM/[Velocity_dot gamma_dot chi_dot] ==
  States : Inport
  Commands : Inport  Port=2
  Gain : Gain  Gain=1/W  SaturateOnIntegerOverflow=on
  Gain2 : Gain  Gain=g  SaturateOnIntegerOverflow=on
  Gain3 : Gain  Gain=g  SaturateOnIntegerOverflow=on
  Math Function : Math  Operator=reciprocal  SaturateOnIntegerOverflow=on
  Subsystem : Subsystem
  Sum1 : Sum  Inputs=|-+  SaturateOnIntegerOverflow=on  InputSameDT=on
  Sum2 : Sum  Inputs=|+-  SaturateOnIntegerOverflow=on  InputSameDT=on
  Sum3 : Sum  Inputs=|+-  SaturateOnIntegerOverflow=on  InputSameDT=on
  "V, gamma, chi1" : BusSelector  OutputSignals=Velocity,loadfactor,gamma,mu
  "V, gamma, chi2" : BusSelector  OutputSignals=Thrust_command
  cos_gamma1 : Trigonometry  Operator=cos
  cos_mu : Trigonometry  Operator=cos
  h_dot1 : Product  SaturateOnIntegerOverflow=on  InputSameDT=on
  h_dot2 : Product  SaturateOnIntegerOverflow=on  InputSameDT=on
  h_dot3 : Product  Inputs=/**  SaturateOnIntegerOverflow=on  InputSameDT=on
  h_dot4 : Product  SaturateOnIntegerOverflow=on  InputSameDT=on
  sin_gamma1 : Trigonometry
  sin_mu : Trigonometry
  Velocity_dot : Outport
  gamma_dot : Outport  Port=2
  chi_dot : Outport  Port=3
  wires:
  "V, gamma, chi1"/1 -> Subsystem/1(Velocity), Math Function/1  "<Velocity>"
  "V, gamma, chi1"/2 -> h_dot2/1, h_dot3/2, Subsystem/2(loadfactor)  "<loadfactor>"
  Subsystem/1(Drag) -> Sum1/1  "Drag"
  Sum1/1 -> Gain/1
  Gain/1 -> Sum2/1
  "V, gamma, chi1"/4 -> cos_mu/1, sin_mu/1  "<mu>"
  sin_gamma1/1 -> Sum2/2
  Sum2/1 -> Gain3/1
  cos_mu/1 -> h_dot2/2
  Math Function/1 -> Gain2/1
  Gain2/1 -> h_dot1/1, h_dot4/1
  h_dot2/1 -> Sum3/1
  cos_gamma1/1 -> Sum3/2, h_dot3/1
  Sum3/1 -> h_dot1/2
  sin_mu/1 -> h_dot3/3
  h_dot3/1 -> h_dot4/2
  States/1 -> "V, gamma, chi1"/1
  Gain3/1 -> Velocity_dot/1  "Velocity_dot"
  h_dot1/1 -> gamma_dot/1  "gamma_dot"
  h_dot4/1 -> chi_dot/1  "chi_dot"
  Commands/1 -> "V, gamma, chi2"/1
  "V, gamma, chi2"/1 -> Sum1/2  "<Thrust_command>"
  "V, gamma, chi1"/3 -> cos_gamma1/1, sin_gamma1/1  "<gamma>"

== system vehicles/Vehicle/EOM/[thrust_dot mu_dot loadfactor_dot] ==
  Comands : Inport
  States : Inport  Port=2
  Constant : Constant  Value=initthis('tau',num_ac);  OutDataType=sfix(16)  ConRadixGroup=Use specified scaling  OutScaling=2^0  SampleTime=inf  FramePeriod=inf
  Matrix Concatenation : Concatenate  NumInputs=3  Mode=Horizontal matrix concatenation
  Matrix Concatenation1 : Concatenate  NumInputs=3  Mode=Horizontal matrix concatenation
  Multiport Selector1 : dspindex/Multiport Selector  rowsOrCols=Columns  idxCellArray={ 1,2,3}  idxErrMode=Clip Index
  Product : Product  Inputs=*/  SaturateOnIntegerOverflow=on  InputSameDT=on
  Reshape : Reshape
  Reshape1 : Reshape
  Reshape2 : Reshape
  Sum : Sum  Inputs=|+-  SaturateOnIntegerOverflow=on  InputSameDT=on
  commands : BusSelector  OutputSignals=Thrust_command,mu_command,loadfactor_command
  thrust,mu,n : BusSelector  OutputSignals=thrust,mu,loadfactor
  thrust_dot : Outport
  mu_dot : Outport  Port=2
  loadfactor_dot : Outport  Port=3
  wires:
  Sum/1 -> Product/1
  Constant/1 -> Product/2
  States/1 -> thrust,mu,n/1
  Comands/1 -> commands/1
  Product/1 -> Multiport Selector1/1  "thrust_dot, mu_dot, loadfactor_dot"
  Multiport Selector1/1 -> Reshape/1
  Multiport Selector1/2 -> Reshape1/1
  Multiport Selector1/3 -> Reshape2/1
  Reshape/1 -> thrust_dot/1  "thrust_dot"
  Reshape1/1 -> mu_dot/1  "mu_dot"
  Reshape2/1 -> loadfactor_dot/1  "loadfactor_dot"
  thrust,mu,n/1 -> Matrix Concatenation/1  "<thrust>"
  thrust,mu,n/2 -> Matrix Concatenation/2  "<mu>"
  thrust,mu,n/3 -> Matrix Concatenation/3  "<loadfactor>"
  Matrix Concatenation/1 -> Sum/2
  commands/1 -> Matrix Concatenation1/1  "<Thrust_command>"
  commands/3 -> Matrix Concatenation1/3  "<loadfactor_command>"
  commands/2 -> Matrix Concatenation1/2  "<mu_command>"
  Matrix Concatenation1/1 -> Sum/1

== system vehicles/Vehicle/EOM/[x_dot y_dot h_dot] ==
  States : Inport
  Product : Product  Inputs=3  SaturateOnIntegerOverflow=on  InputSameDT=on
  Product1 : Product  SaturateOnIntegerOverflow=on  InputSameDT=on
  Product2 : Product  Inputs=3  SaturateOnIntegerOverflow=on  InputSameDT=on
  "V, gamma, chi" : BusSelector  OutputSignals=Velocity,gamma,chi
  cos_chi : Trigonometry  Operator=cos
  cos_gamma : Trigonometry  Operator=cos
  sin_chi : Trigonometry
  sin_gamma : Trigonometry
  x_dot : Outport
  y_dot : Outport  Port=2
  h_dot : Outport  Port=3
  wires:
  "V, gamma, chi"/1 -> Product2/1, Product/1, Product1/1  "<Velocity>"
  "V, gamma, chi"/2 -> sin_gamma/1, cos_gamma/1  "<gamma>"
  "V, gamma, chi"/3 -> sin_chi/1, cos_chi/1  "<chi>"
  cos_gamma/1 -> Product2/2, Product/2
  cos_chi/1 -> Product2/3
  sin_chi/1 -> Product/3
  sin_gamma/1 -> Product1/2
  States/1 -> "V, gamma, chi"/1
  Product2/1 -> x_dot/1  "x_dot"
  Product/1 -> y_dot/1  "y_dot"
  Product1/1 -> h_dot/1  "h_dot"

== system vehicles/Instincts/Collabrative Instincts/AC avoidance instinct calculations/Distance between AC Calculator1 ==
  note: The output of this FOR system should be a diagonal symetric matrix
      | I am doing twice as many calculations as needed.  Maybe I'll get rid
      | of that someday.
  num_ac : Inport
  positions : Inport  Port=2
  initial matrix : Inport  Port=3
  Assignment : Assignment  InputType=Matrix  IndexIsStartValue=off  ElementSrc=External  Elements=1  RowSrc=External  Rows=1  ColumnSrc=External  Columns=1  OutputDimensions=[1 1]
  Constant : Constant  Value=[1:num_ac]  OutDataType=sfix(16)  ConRadixGroup=Use specified scaling  OutScaling=2^0  SampleTime=inf  FramePeriod=inf
  For Iterator : ForIterator  IterationSource=external  IterationVariableDataType=double
  For Iterator Subsystem : Subsystem  TreatAsAtomicUnit=on
  Ground : Ground
  Selector : Selector  InputType=Matrix  ElementSrc=Internal  Elements=[1 3]  RowSrc=External  Rows=1  ColumnSrc=Internal  Columns=-1  InputPortWidth=3  IndexIsStartValue=off
  Signal Specification : SignalSpecification  Dimensions=[1,num_ac]
  Distance matrix : Outport
  wires:
  num_ac/1 -> For Iterator/1, For Iterator Subsystem/1(num_ac)
  For Iterator/1 -> Selector/2, For Iterator Subsystem/5(row), Assignment/3
  positions/1 -> Selector/1, For Iterator Subsystem/2(positions)
  Selector/1 -> For Iterator Subsystem/3(position)
  For Iterator Subsystem/1(row for one aircraft) -> Assignment/2
  Ground/1 -> Signal Specification/1
  Signal Specification/1 -> For Iterator Subsystem/4(initial row)
  initial matrix/1 -> Assignment/1
  Assignment/1 -> Distance matrix/1
  Constant/1 -> Assignment/4

== system vehicles/Instincts/Collabrative Instincts/AC avoidance instinct calculations/normalize across rows ==
  note: change above to column sum if you
      | want to normalize across columns
  In1 : Inport
  Math Function : Math  Operator=square  SaturateOnIntegerOverflow=on
  Math Function1 : Math  Operator=sqrt  SaturateOnIntegerOverflow=on
  Math Function2 : Math  Operator=reciprocal  SaturateOnIntegerOverflow=on
  Matrix Scaling : dspmtrx3/Matrix Scaling  DialogController=dspDDGCreate  DialogControllerArgs=DataTag3  mode=Scale rows (D*A)  D_Source=Input port  D_VectFromMask=[0.5 0.25]  roundingMode=Floor  overflowMode=off
  Matrix Sum : dspmtrx3/Matrix Sum  DialogController=dspDDGCreate  DialogControllerArgs=DataTag4  Dim=Rows  roundingMode=Floor  overflowMode=off
  Out1 : Outport
  wires:
  In1/1 -> Matrix Scaling/1, Math Function/1
  Math Function/1 -> Matrix Sum/1
  Matrix Sum/1 -> Math Function1/1
  Math Function1/1 -> Math Function2/1
  Math Function2/1 -> Matrix Scaling/2
  Matrix Scaling/1 -> Out1/1

== system vehicles/Instincts/Collabrative Instincts/formation keeping instinct calculations/normalize across rows ==
  In1 : Inport
  Math Function : Math  Operator=square  SaturateOnIntegerOverflow=on
  Math Function1 : Math  Operator=sqrt  SaturateOnIntegerOverflow=on
  Math Function2 : Math  Operator=reciprocal  SaturateOnIntegerOverflow=on
  Matrix Scaling : dspmtrx3/Matrix Scaling  DialogController=dspDDGCreate  DialogControllerArgs=DataTag5  mode=Scale rows (D*A)  D_Source=Input port  D_VectFromMask=[0.5 0.25]  roundingMode=Floor  overflowMode=off
  Matrix Sum : dspmtrx3/Matrix Sum  DialogController=dspDDGCreate  DialogControllerArgs=DataTag6  Dim=Rows  roundingMode=Floor  overflowMode=off
  Out1 : Outport
  wires:
  In1/1 -> Matrix Scaling/1, Math Function/1
  Math Function/1 -> Matrix Sum/1
  Matrix Sum/1 -> Math Function1/1
  Math Function1/1 -> Math Function2/1
  Math Function2/1 -> Matrix Scaling/2
  Matrix Scaling/1 -> Out1/1

== system vehicles/Instincts/Collabrative Instincts/obstacle avoidance instinct calculations/Angle calulator ==
  States : Inport
  position_to_closest_obs : Inport  Port=2
  Extract Diagonal : dspmtrx3/Extract Diagonal
  Matrix Multiply : Product  Multiplication=Matrix(*)
  Transpose1 : dspmtrx3/Transpose  SystemSampleTime=-1  Hermitian=off  overflowFlag=on
  Trigonometric Function : Trigonometry  Operator=acos
  "[x_dot y_dot h_dot]" : Subsystem
  normalize across rows : Subsystem
  normalize across rows1 : Subsystem
  velocity vectors of each AC : Concatenate  NumInputs=3  Mode=Horizontal matrix concatenation
  angle_between_velvec_obsvec : Outport
  wires:
  "[x_dot y_dot h_dot]"/3(h_dot) -> velocity vectors of each AC/3
  "[x_dot y_dot h_dot]"/2(y_dot) -> velocity vectors of each AC/2
  "[x_dot y_dot h_dot]"/1(x_dot) -> velocity vectors of each AC/1
  velocity vectors of each AC/1 -> normalize across rows/1(In1)
  normalize across rows/1(Out1) -> Matrix Multiply/1
  normalize across rows1/1(Out1) -> Transpose1/1
  Transpose1/1 -> Matrix Multiply/2
  Matrix Multiply/1 -> Extract Diagonal/1
  Extract Diagonal/1 -> Trigonometric Function/1
  States/1 -> "[x_dot y_dot h_dot]"/1(States)
  Trigonometric Function/1 -> angle_between_velvec_obsvec/1
  position_to_closest_obs/1 -> normalize across rows1/1(In1)

== system vehicles/Instincts/Collabrative Instincts/obstacle avoidance instinct calculations/Distance from obstacles Calculator ==
  num_ac : Inport
  position of ac : Inport  Port=2
  initial matrix : Inport  Port=3
  Assignment : Assignment  InputType=Matrix  IndexIsStartValue=off  ElementSrc=External  Elements=1  RowSrc=External  Rows=1  ColumnSrc=External  Columns=1  OutputDimensions=[1 1]
  Constant : Constant  Value=[1:size(obstacles.positions,1)]  OutDataType=sfix(16)  ConRadixGroup=Use specified scaling  OutScaling=2^0  SampleTime=inf  FramePeriod=inf
  Constant1 : Constant  Value=obstacles.positions  OutDataType=sfix(16)  ConRadixGroup=Use specified scaling  OutScaling=2^0  SampleTime=inf  FramePeriod=inf
  Constant2 : Constant  Value=size(obstacles.positions,1)  OutDataType=sfix(16)  ConRadixGroup=Use specified scaling  OutScaling=2^0  SampleTime=inf  FramePeriod=inf
  For Iterator : ForIterator  IterationSource=external  IterationVariableDataType=double
  For Iterator Subsystem : Subsystem  TreatAsAtomicUnit=on
  Ground : Ground
  Selector : Selector  InputType=Matrix  ElementSrc=Internal  Elements=[1 3]  RowSrc=External  Rows=1  ColumnSrc=Internal  Columns=-1  InputPortWidth=3  IndexIsStartValue=off
  Signal Specification : SignalSpecification  Dimensions=[size(obstacles.positions,1),1]
  Distance matrix : Outport
  wires:
  num_ac/1 -> For Iterator/1
  For Iterator/1 -> Selector/2, Assignment/4
  position of ac/1 -> Selector/1
  Selector/1 -> For Iterator Subsystem/3(position of ac)
  For Iterator Subsystem/1(row for one obstacle) -> Assignment/2
  Ground/1 -> Signal Specification/1
  Signal Specification/1 -> For Iterator Subsystem/4(initial column)
  initial matrix/1 -> Assignment/1
  Assignment/1 -> Distance matrix/1
  Constant1/1 -> For Iterator Subsystem/1(position of obs)
  Constant/1 -> Assignment/3
  Constant2/1 -> For Iterator Subsystem/2(num_obs)

== system vehicles/Instincts/Collabrative Instincts/obstacle avoidance instinct calculations/LOS Angle calculator ==
  closest_obs_distmag : Inport
  closest_obs_ind : Inport  Port=2
  Constant2 : Constant  Value=obstacles.radius  OutDataType=sfix(16)  ConRadixGroup=Use specified scaling  OutScaling=2^0  SampleTime=inf  FramePeriod=inf
  Gain : Gain  Gain=2  SaturateOnIntegerOverflow=on
  Product : Product  Inputs=*/  SaturateOnIntegerOverflow=on  InputSameDT=on
  Trigonometric Function1 : Trigonometry  Operator=atan
  radius of closest object vecor : Selector  InputType=Vector  ElementSrc=External  Elements=[1 3]  RowSrc=External  Rows=1  ColumnSrc=Internal  Columns=-1  IndexIsStartValue=off
  los_angle_between_obs_edges : Outport
  wires:
  radius of closest object vecor/1 -> Product/1
  Product/1 -> Trigonometric Function1/1
  Trigonometric Function1/1 -> Gain/1
  Gain/1 -> los_angle_between_obs_edges/1
  closest_obs_distmag/1 -> Product/2
  closest_obs_ind/1 -> radius of closest object vecor/2
  Constant2/1 -> radius of closest object vecor/1
